simulink model "switch_temp3"  (Simulink 7.8)
settings: Solver=ode45  StartTime=0.0  StopTime=4  RelTol=1e-3
values from neighbouring files (symbols this model uses):
  A1 = [0 1 ; -1 -2]    [switch_test1.m]
undefined symbols (not defined in the file or in its folder): A2, B1, B2, C1, C2, D1, D2
libraries: simulink x2
settings Model: Creator=rpichard  LastModifiedBy=rpichard

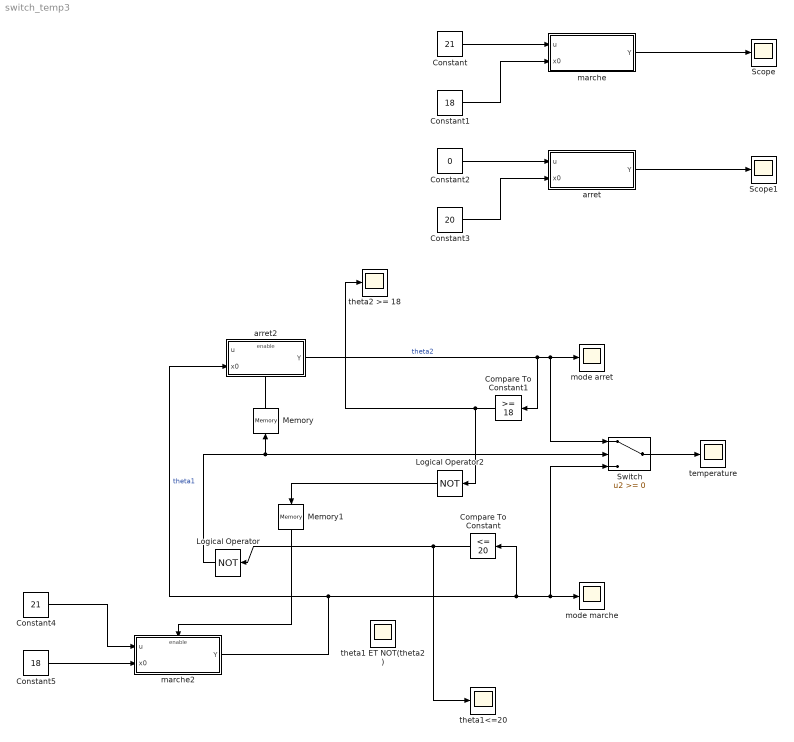
== system switch_temp3 ==
  Compare To Constant : simulink/Logic and Bit Operations/Compare To Constant  relop=<=  const=20  OutDataTypeStr=boolean  ZeroCross=off
  Compare To Constant1 : simulink/Logic and Bit Operations/Compare To Constant  relop=>=  const=18  OutDataTypeStr=boolean  ZeroCross=off
  Constant : Constant  Value=21
  Constant1 : Constant  Value=18
  Constant2 : Constant  Value=0
  Constant3 : Constant  Value=20
  Constant4 : Constant  Value=21
  Constant5 : Constant  Value=18
  Logical Operator : Logic  Operator=NOT  AllPortsSameDT=off  OutDataTypeStr=boolean
  Logical Operator2 : Logic  Operator=NOT  AllPortsSameDT=off  OutDataTypeStr=boolean
  Memory : Memory
  Memory1 : Memory
  Scope : Scope
  Scope1 : Scope
  Switch : Switch  RequirementInfo="{}  %GIDa_b5fc659a_16ec_4afa_8660_c5a00df90d5b"
  arret : Subsystem
  arret2 : Subsystem  TreatAsAtomicUnit=on
  marche : Subsystem
  marche2 : Subsystem  TreatAsAtomicUnit=on
  mode arret : Scope
      settings: SaveName=ScopeData4
  mode marche : Scope
      settings: TimeRange=4  SaveName=ScopeData3
  temperature : Scope
      settings: SaveName=ScopeData5
  theta1 ET NOT(theta2) : Scope
      settings: SaveName=ScopeData7
  theta1<=20 : Scope
      settings: SaveName=ScopeData6
  theta2 >= 18 : Scope
      settings: SaveName=ScopeData2
  wires:
  Constant/1 -> marche/1(u)
  Constant1/1 -> marche/2(x0)
  marche/1(Y) -> Scope/1
  Constant2/1 -> arret/1(u)
  Constant3/1 -> arret/2(x0)
  arret/1(Y) -> Scope1/1
  marche2/1(Y) -> Compare To Constant/1, Switch/3, mode marche/1, arret2/2(x0)  "theta1"
  Constant4/1 -> marche2/1(u)
  Constant5/1 -> marche2/2(x0)
  Logical Operator/1 -> Switch/2, Memory/1
  arret2/1(Y) -> mode arret/1, Switch/1, Compare To Constant1/1  "theta2"
  Switch/1 -> temperature/1
  Compare To Constant1/1 -> theta2 >= 18/1, Logical Operator2/1
  Compare To Constant/1 -> theta1<=20/1, Logical Operator/1
  Memory/1 -> arret2/Enable
  Logical Operator2/1 -> Memory1/1
  Memory1/1 -> marche2/Enable

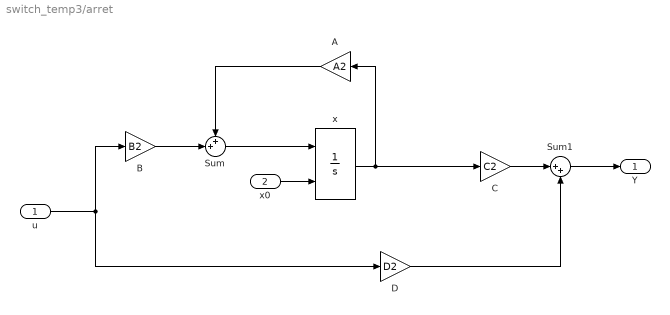
== system switch_temp3/arret ==
  u : Inport
  x0 : Inport  Port=2
  A : Gain  Gain=A2
  B : Gain  Gain=B2
  C : Gain  Gain=C2
  D : Gain  Gain=D2
  Sum : Sum  Inputs=++|
  Sum1 : Sum  Inputs=|++
  x : Integrator  InitialConditionSource=external
  Y : Outport
  wires:
  x/1 -> A/1, C/1
  Sum/1 -> x/1
  A/1 -> Sum/1
  x0/1 -> x/2
  u/1 -> D/1, B/1
  C/1 -> Sum1/1
  Sum1/1 -> Y/1
  D/1 -> Sum1/2
  B/1 -> Sum/2

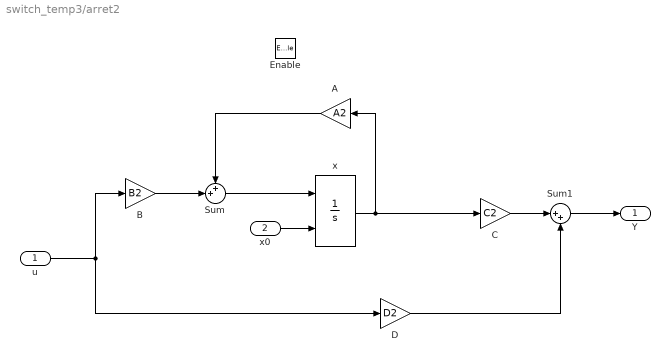
== system switch_temp3/arret2 ==
  u : Inport
  x0 : Inport  Port=2
  Enable : EnablePort  StatesWhenEnabling=reset
  A : Gain  Gain=A2
  B : Gain  Gain=B2
  C : Gain  Gain=C2
  D : Gain  Gain=D2
  Sum : Sum  Inputs=++|
  Sum1 : Sum  Inputs=|++
  x : Integrator  InitialConditionSource=external
  Y : Outport
  wires:
  x/1 -> A/1, C/1
  Sum/1 -> x/1
  A/1 -> Sum/1
  x0/1 -> x/2
  u/1 -> D/1, B/1
  C/1 -> Sum1/1
  Sum1/1 -> Y/1
  D/1 -> Sum1/2
  B/1 -> Sum/2

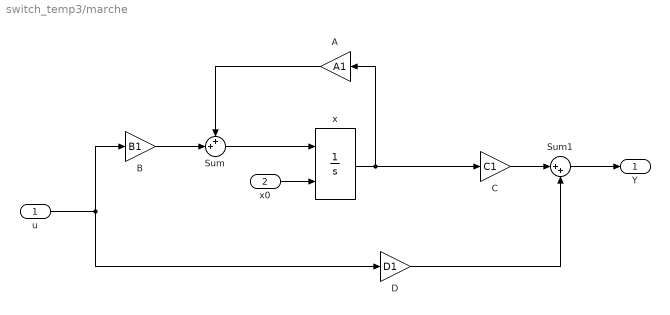
== system switch_temp3/marche ==
  u : Inport
  x0 : Inport  Port=2
  A : Gain  Gain=A1
  B : Gain  Gain=B1
  C : Gain  Gain=C1
  D : Gain  Gain=D1
  Sum : Sum  Inputs=++|
  Sum1 : Sum  Inputs=|++
  x : Integrator  InitialConditionSource=external
  Y : Outport
  wires:
  x/1 -> A/1, C/1
  Sum/1 -> x/1
  A/1 -> Sum/1
  x0/1 -> x/2
  u/1 -> D/1, B/1
  C/1 -> Sum1/1
  Sum1/1 -> Y/1
  D/1 -> Sum1/2
  B/1 -> Sum/2

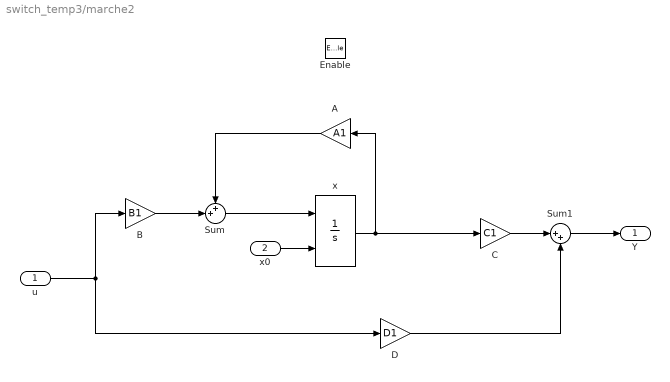
== system switch_temp3/marche2 ==
  u : Inport
  x0 : Inport  Port=2
  Enable : EnablePort  StatesWhenEnabling=reset
  A : Gain  Gain=A1
  B : Gain  Gain=B1
  C : Gain  Gain=C1
  D : Gain  Gain=D1
  Sum : Sum  Inputs=++|
  Sum1 : Sum  Inputs=|++
  x : Integrator  InitialConditionSource=external
  Y : Outport
  wires:
  x/1 -> A/1, C/1
  Sum/1 -> x/1
  A/1 -> Sum/1
  x0/1 -> x/2
  u/1 -> D/1, B/1
  C/1 -> Sum1/1
  Sum1/1 -> Y/1
  D/1 -> Sum1/2
  B/1 -> Sum/2
